simulink model "Message_eg"  (R2018a)
settings: Solver=VariableStepAuto  StartTime=0.0  StopTime=10.0  RelTol=1e-3
settings Model: Creator=86188  LastModifiedBy=86188

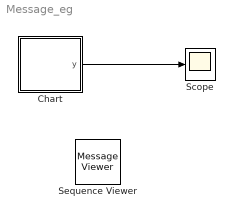
== system Message_eg ==
  Chart : Stateflow chart  TreatAsAtomicUnit=on
  Scope : Scope
  Sequence Viewer : MessageViewer
  wires:
  Chart/1(y) -> Scope/1

== stateflow chart Message_eg/Chart ==
  state A
    en:
    M.data=3;
    send(M);
  state B
    y=1;
  (default) -> A
  A -> B : M[M.data==3]
  data: M local; y output
